simulink model "ex8impnmpc6"  (R2025b)
settings: Solver=VariableStepAuto  StartTime=0.0  StopTime=8000  RelTol=1e-3
values from neighbouring files (symbols this model uses):
  K = nmpc_design_st2(par)    [ex16.m]    (also in ex26.m; ex46.m)
  ref = [6971 0 0 0 0]    [ex16.m]    (also in ex26.m = [9192.3, 0.22, 0.026, 0, 0]; ex46.m = [0;0])
  x0 = [rp;vp]    [ex1.m]    (also in ex13.m = [randi([-i,1]),randi([0,i])]; ex16.m = [rp;vp;mb+mp0]; ex21.m = [0.31156,0.23895,0.2768]; ex22.m = [randi([-2,2]),randi([-4,4])])
undefined symbols (not defined in the file or in its folder): rv2oe, spacecraft_dynamics
settings Model: Creator=Esteban  LastModifiedBy=Esteban

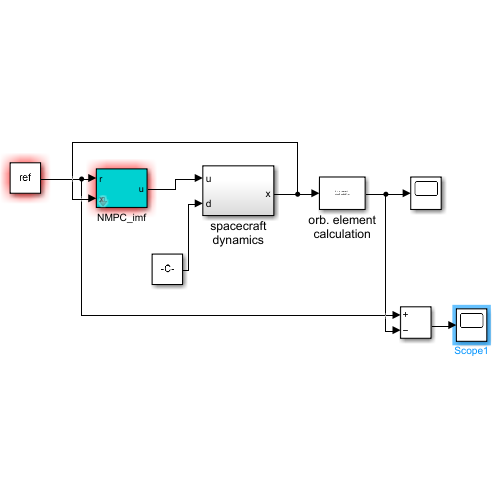
[thumbnail: Simulink's stored preview of the top-level diagram]
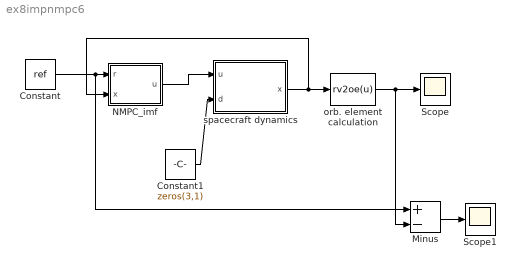
== system ex8impnmpc6 ==
  Constant : Constant  Value=ref
  Constant1 : Constant  Value=zeros(3,1)
  Minus : Sum  Inputs=+-
  NMPC_imf : Subsystem  mask{K=K}
      mask prompts: K "NMPC structure"
  Scope : Scope
  Scope1 : Scope
      settings: ActiveDisplayYMinimum=-573.28970613029287  ActiveDisplayYMaximum=262.23297736183582
  orb. element calculation : MATLABFcn  MATLABFcn=rv2oe(u)  OutputDimensions=5
  spacecraft dynamics : Subsystem
  wires:
  Constant/1 -> Minus/1, NMPC_imf/1(r)
  NMPC_imf/1(u) -> spacecraft dynamics/1(u)
  Constant1/1 -> spacecraft dynamics/2(d)
  spacecraft dynamics/1(x) -> NMPC_imf/2(x), orb. element calculation/1
  orb. element calculation/1 -> Minus/2, Scope/1
  Minus/1 -> Scope1/1

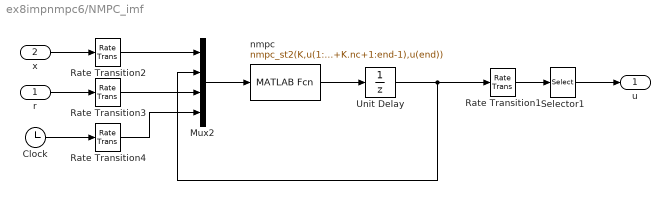
== system ex8impnmpc6/NMPC_imf ==
  r : Inport
  x : Inport  Port=2
  Clock : Clock
  Mux2 : Mux
  Rate Transition{1..4} (4 alike) : RateTransition  OutPortSampleTime=K.Ts
  Selector1 : Selector  InputPortWidth=K.nc  IndexOptions=Index vector (dialog)  Indices=1:K.nu  OutputSizes=1
  Unit Delay : UnitDelay  InitialCondition=zeros(K.nc,1)  SampleTime=K.Ts  HasFrameUpgradeWarning=on
  nmpc : MATLABFcn  MATLABFcn=nmpc_st2(K,u(1:K.nx),u(K.nx+1:K.nx+K.nc),u(K.nx+K.nc+1:end-1),u(end))  OutputDimensions=K.nc
  u : Outport  PortDimensions=K.nu
  wires:
  x/1 -> Rate Transition2/1
  Unit Delay/1 -> Rate Transition1/1, Mux2/2
  Mux2/1 -> nmpc/1
  r/1 -> Rate Transition3/1
  Rate Transition2/1 -> Mux2/1
  Rate Transition1/1 -> Selector1/1
  Rate Transition3/1 -> Mux2/3
  nmpc/1 -> Unit Delay/1
  Selector1/1 -> u/1
  Clock/1 -> Rate Transition4/1
  Rate Transition4/1 -> Mux2/4

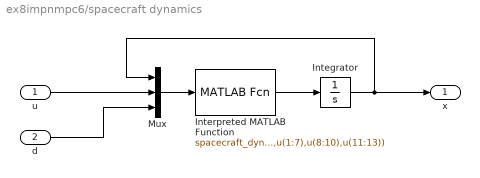
== system ex8impnmpc6/spacecraft dynamics ==
  u : Inport
  d : Inport  Port=2
  Integrator : Integrator  InitialCondition=x0
  Interpreted MATLAB Function : MATLABFcn  MATLABFcn=spacecraft_dynamics(0,u(1:7),u(8:10),u(11:13))
  Mux : Mux  Inputs=3
  x : Outport  VectorParamsAs1DForOutWhenUnconnected=off
  wires:
  Mux/1 -> Interpreted MATLAB Function/1
  Integrator/1 -> Mux/1, x/1
  Interpreted MATLAB Function/1 -> Integrator/1
  u/1 -> Mux/2
  d/1 -> Mux/3
